simulink model "L400_airframe_test"  (R2024b)
settings: Solver=FixedStepAuto  StartTime=0.0  StopTime=100  FixedStep=0.005  RelTol=1e-3
libraries: simulink x1
settings Model: DataDictionary=nextpilot_datadict.sldd  Creator=CETCA  LastModifiedBy=CETCA

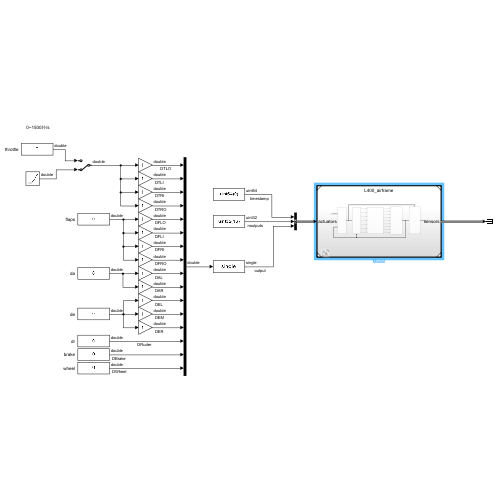
[thumbnail: Simulink's stored preview of the top-level diagram]
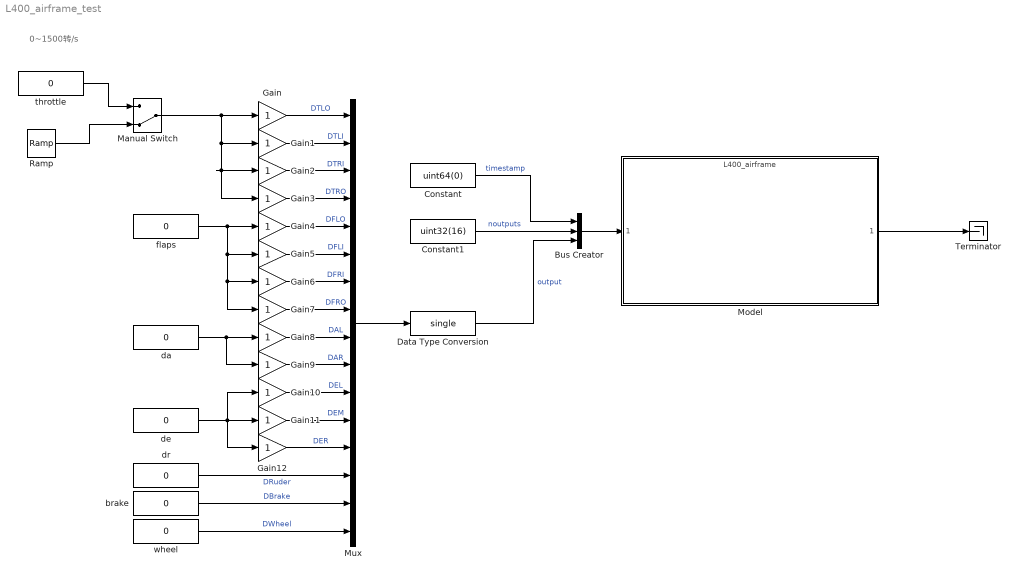
== system L400_airframe_test ==
  note: 0~1500转/s
  Bus Creator : BusCreator  Inputs=3
  Constant : Constant  Value=uint64(0)
  Constant1 : Constant  Value=uint32(16)
  Data Type Conversion : DataTypeConversion  OutDataTypeStr=single  SaturateOnIntegerOverflow=off  RndMeth=Floor
  Gain{,1..12} (13 alike) : Gain
  Manual Switch : ManualSwitch  CurrentSetting=0
  Model : ModelReference  ModelNameDialog=L400_airframe.slx  SimulationMode=Normal  ModelReferenceVersion=5.334
  Mux : Mux  Inputs=16
  Ramp : simulink/Sources/Ramp  slope=10  start=5  InitialOutput=0
  Terminator : Terminator
  brake : Constant  Value=0
  da : Constant  Value=0
  de : Constant  Value=0
  dr : Constant  Value=0
  flaps : Constant  Value=0
  throttle : Constant  Value=0
  wheel : Constant  Value=0
  wires:
  Manual Switch/1 -> Gain1/1, Gain3/1, Gain2/1, Gain/1
  Bus Creator/1 -> Model/1
  Constant/1 -> Bus Creator/1  "timestamp"
  Mux/1 -> Data Type Conversion/1
  de/1 -> Gain12/1, Gain10/1, Gain11/1
  Constant1/1 -> Bus Creator/2  "noutputs"
  flaps/1 -> Gain7/1, Gain6/1, Gain5/1, Gain4/1
  Data Type Conversion/1 -> Bus Creator/3  "output"
  da/1 -> Gain8/1, Gain9/1
  Gain/1 -> Mux/1  "DTLO"
  Gain1/1 -> Mux/2  "DTLI"
  Gain2/1 -> Mux/3  "DTRI"
  Gain3/1 -> Mux/4  "DTRO"
  Gain4/1 -> Mux/5  "DFLO"
  Gain5/1 -> Mux/6  "DFLI"
  Gain6/1 -> Mux/7  "DFRI"
  Gain7/1 -> Mux/8  "DFRO"
  Gain8/1 -> Mux/9  "DAL"
  Gain9/1 -> Mux/10  "DAR"
  Gain10/1 -> Mux/11  "DEL"
  Gain11/1 -> Mux/12  "DEM"
  Gain12/1 -> Mux/13  "DER"
  dr/1 -> Mux/14  "DRuder"
  brake/1 -> Mux/15  "DBrake"
  wheel/1 -> Mux/16  "DWheel"
  Model/1 -> Terminator/1
  throttle/1 -> Manual Switch/1
  Ramp/1 -> Manual Switch/2
